simulink model "singlcontact_control_smc_lqr_mydimes_reaction"  (R2024a)
settings: Solver=VariableStepAuto  StartTime=0.0  StopTime=10  FixedStep=0.001  RelTol=1e-3
values from neighbouring files (symbols this model uses):
  ankle_servo_kd = 8    [robotParametersCtrl_mydiem_block_zmp.m]    (also in robotParametersCtrl_quad_modify_mydiem.m; robotParametersCtrl_quad_modify_mydiem_reaction.m)
  ankle_servo_ki = 4    [robotParametersCtrl_mydiem_block_zmp.m]    (also in robotParametersCtrl_quad_modify_mydiem.m; robotParametersCtrl_quad_modify_mydiem_reaction.m)
  ankle_servo_kp = 20    [robotParametersCtrl_mydiem_block_zmp.m]    (also in robotParametersCtrl_quad_modify_mydiem.m; robotParametersCtrl_quad_modify_mydiem_reaction.m)
  deriv_filter_coeff = 100    [robotParametersCtrl_mydiem_block_zmp.m]    (also in robotParametersCtrl_quad_modify_mydiem.m; robotParametersCtrl_quad_modify_mydiem_reaction.m)
  filter_coefficent_pid = 100    [robotParametersCtrl_mydiem_block_zmp.m]    (also in robotParametersCtrl_quad_modify_mydiem.m; robotParametersCtrl_quad_modify_mydiem_reaction.m)
  filter_coefficent_pids = 100    [robotParametersCtrl_quad_modify_mydiem_reaction.m]
  foot_z = 1.5    [robotParametersCtrl_mydiem_block_zmp.m]    (also in robotParametersCtrl_quad_modify_mydiem.m; robotParametersCtrl_quad_modify_mydiem_reaction.m)
  g = 9.81    [ABCDvalues_lqr_quad_mydime_reaction.m]    (also in robotParametersCtrl_mydiem_block_zmp.m = 9.80665; robotParametersCtrl_quad_modify_mydiem.m = 9.80665; robotParametersCtrl_quad_modify_mydiem_reaction.m = 9.80665)
  h = 32    [robotParametersCtrl_mydiem_block_zmp.m]    (also in robotParametersCtrl_quad_modify_mydiem.m; robotParametersCtrl_quad_modify_mydiem_reaction.m)
  height_plane = 0.025    [robotParametersCtrl_mydiem_block_zmp.m]    (also in robotParametersCtrl_quad_modify_mydiem.m; robotParametersCtrl_quad_modify_mydiem_reaction.m)
  hip_pitch_deriv = 20    [robotParametersCtrl_mydiem_block_zmp.m]    (also in robotParametersCtrl_quad_modify_mydiem.m = 200; robotParametersCtrl_quad_modify_mydiem_reaction.m = 200)
  hip_pitch_derivs = 200    [robotParametersCtrl_quad_modify_mydiem_reaction.m]
  hip_pitch_int = 0    [robotParametersCtrl_mydiem_block_zmp.m]    (also in robotParametersCtrl_quad_modify_mydiem.m = 150; robotParametersCtrl_quad_modify_mydiem_reaction.m = 150)
  hip_pitch_ints = 1500    [robotParametersCtrl_quad_modify_mydiem_reaction.m]
  hip_pitch_prop = 10    [robotParametersCtrl_mydiem_block_zmp.m]    (also in robotParametersCtrl_quad_modify_mydiem.m = 500; robotParametersCtrl_quad_modify_mydiem_reaction.m = 500)
  hip_pitch_props = 500    [robotParametersCtrl_quad_modify_mydiem_reaction.m]
  hip_roll_deriv = 28    [robotParametersCtrl_mydiem_block_zmp.m]    (also in robotParametersCtrl_quad_modify_mydiem.m = 280; robotParametersCtrl_quad_modify_mydiem_reaction.m = 280)
  hip_roll_derivs = 280    [robotParametersCtrl_quad_modify_mydiem_reaction.m]
  hip_roll_int = 0    [robotParametersCtrl_mydiem_block_zmp.m]    (also in robotParametersCtrl_quad_modify_mydiem.m = 180; robotParametersCtrl_quad_modify_mydiem_reaction.m = 180)
  hip_roll_ints = 180    [robotParametersCtrl_quad_modify_mydiem_reaction.m]
  hip_roll_prop = 10    [robotParametersCtrl_mydiem_block_zmp.m]    (also in robotParametersCtrl_quad_modify_mydiem.m = 300; robotParametersCtrl_quad_modify_mydiem_reaction.m = 300)
  hip_roll_props = 300    [robotParametersCtrl_quad_modify_mydiem_reaction.m]
  hip_servo_kd = 20    [robotParametersCtrl_mydiem_block_zmp.m]    (also in robotParametersCtrl_quad_modify_mydiem.m; robotParametersCtrl_quad_modify_mydiem_reaction.m)
  hip_servo_ki = 10    [robotParametersCtrl_mydiem_block_zmp.m]    (also in robotParametersCtrl_quad_modify_mydiem.m; robotParametersCtrl_quad_modify_mydiem_reaction.m)
  hip_servo_kp = 60    [robotParametersCtrl_mydiem_block_zmp.m]    (also in robotParametersCtrl_quad_modify_mydiem.m; robotParametersCtrl_quad_modify_mydiem_reaction.m)
  hip_smc_lamda = 85    [robotParametersCtrl_mydiem_block_zmp.m]    (also in robotParametersCtrl_quad_modify_mydiem.m; robotParametersCtrl_quad_modify_mydiem_reaction.m = 95)
  hip_smc_lamdas = 85    [robotParametersCtrl_quad_modify_mydiem_reaction.m]
  hip_smc_new = 25    [robotParametersCtrl_mydiem_block_zmp.m]    (also in robotParametersCtrl_quad_modify_mydiem.m; robotParametersCtrl_quad_modify_mydiem_reaction.m = 45)
  hip_smc_news = 25    [robotParametersCtrl_quad_modify_mydiem_reaction.m]
  init_angs_L = init_angs_R    [robotParametersCtrl_mydiem_block_zmp.m]    (also in robotParametersCtrl_quad_modify_mydiem.m; robotParametersCtrl_quad_modify_mydiem_reaction.m)
  init_angs_R = [0 -sum(init_angs) init_angs(2) 0 init_angs(1)]    [robotParametersCtrl_mydiem_block_zmp.m]    (also in robotParametersCtrl_quad_modify_mydiem.m; robotParametersCtrl_quad_modify_mydiem_reaction.m)
  init_height = h +                torso_z/2 + torso_offset_z + height_plane/2    (= 39.5125)    [robotParametersCtrl_mydiem_block_zmp.m]    (also in robotParametersCtrl_quad_modify_mydiem.m; robotParametersCtrl_quad_modify_mydiem_reaction.m)
  K = lqr(A, B, Q, R)    [ABCDvalues_lqr_quad_mydime_reaction.m]
  knee_pitch_deriv = 10    [robotParametersCtrl_mydiem_block_zmp.m]    (also in robotParametersCtrl_quad_modify_mydiem.m = 100; robotParametersCtrl_quad_modify_mydiem_reaction.m = 100)
  knee_pitch_derivs = 180    [robotParametersCtrl_quad_modify_mydiem_reaction.m]
  knee_pitch_int = 0    [robotParametersCtrl_mydiem_block_zmp.m]    (also in robotParametersCtrl_quad_modify_mydiem.m = 300; robotParametersCtrl_quad_modify_mydiem_reaction.m = 300)
  knee_pitch_ints = 7500    [robotParametersCtrl_quad_modify_mydiem_reaction.m]
  knee_pitch_prop = 10    [robotParametersCtrl_mydiem_block_zmp.m]    (also in robotParametersCtrl_quad_modify_mydiem.m = 400; robotParametersCtrl_quad_modify_mydiem_reaction.m = 400)
  knee_pitch_props = 1200    [robotParametersCtrl_quad_modify_mydiem_reaction.m]
  knee_servo_kd = 10    [robotParametersCtrl_mydiem_block_zmp.m]    (also in robotParametersCtrl_quad_modify_mydiem.m; robotParametersCtrl_quad_modify_mydiem_reaction.m)
  knee_servo_ki = 5    [robotParametersCtrl_mydiem_block_zmp.m]    (also in robotParametersCtrl_quad_modify_mydiem.m; robotParametersCtrl_quad_modify_mydiem_reaction.m)
  knee_servo_kp = 60    [robotParametersCtrl_mydiem_block_zmp.m]    (also in robotParametersCtrl_quad_modify_mydiem.m; robotParametersCtrl_quad_modify_mydiem_reaction.m)
  knee_smc_lamda = 140    [robotParametersCtrl_mydiem_block_zmp.m]    (also in robotParametersCtrl_quad_modify_mydiem.m; robotParametersCtrl_quad_modify_mydiem_reaction.m = 150)
  knee_smc_lamdas = 100    [robotParametersCtrl_quad_modify_mydiem_reaction.m]
  knee_smc_new = 80    [robotParametersCtrl_mydiem_block_zmp.m]    (also in robotParametersCtrl_quad_modify_mydiem.m; robotParametersCtrl_quad_modify_mydiem_reaction.m)
  knee_smc_news = 60    [robotParametersCtrl_quad_modify_mydiem_reaction.m]
  Kwalk = 0.6    [robotParametersCtrl_mydiem_block_zmp.m]    (also in robotParametersCtrl_quad_modify_mydiem.m; robotParametersCtrl_quad_modify_mydiem_reaction.m)
  l1 = 0.20    (= 0.2)    [ABCDvalues_lqr_quad_mydime_reaction.m]
  l2 = 0.20    (= 0.2)    [ABCDvalues_lqr_quad_mydime_reaction.m]
  lower_leg_length = 20    [robotParametersCtrl_mydiem_block_zmp.m]    (also in robotParametersCtrl_quad_modify_mydiem.m; robotParametersCtrl_quad_modify_mydiem_reaction.m)
  m1 = 0.45    [ABCDvalues_lqr_quad_mydime_reaction.m]
  m2 = 0.065    [ABCDvalues_lqr_quad_mydime_reaction.m]
  max_torque = 20    [robotParametersCtrl_mydiem_block_zmp.m]    (also in robotParametersCtrl_quad_modify_mydiem.m; robotParametersCtrl_quad_modify_mydiem_reaction.m)
  motion_time_constant = 0.01    [robotParametersCtrl_mydiem_block_zmp.m]    (also in robotParametersCtrl_quad_modify_mydiem.m; robotParametersCtrl_quad_modify_mydiem_reaction.m)
  plane_x = 25    [robotParametersCtrl_mydiem_block_zmp.m]    (also in robotParametersCtrl_quad_modify_mydiem.m; robotParametersCtrl_quad_modify_mydiem_reaction.m)
  plane_y = 3    [robotParametersCtrl_mydiem_block_zmp.m]    (also in robotParametersCtrl_quad_modify_mydiem.m; robotParametersCtrl_quad_modify_mydiem_reaction.m)
  stepHeight = 0.4    [ABCDvalues_lqr_quad_mydime_reaction.m]
  torso_offset_x = 17    [robotParametersCtrl_mydiem_block_zmp.m]    (also in robotParametersCtrl_quad_modify_mydiem.m; robotParametersCtrl_quad_modify_mydiem_reaction.m)
  torso_offset_x1 = -17    [robotParametersCtrl_mydiem_block_zmp.m]    (also in robotParametersCtrl_quad_modify_mydiem.m; robotParametersCtrl_quad_modify_mydiem_reaction.m)
  torso_offset_z = 0    [robotParametersCtrl_mydiem_block_zmp.m]    (also in robotParametersCtrl_quad_modify_mydiem.m; robotParametersCtrl_quad_modify_mydiem_reaction.m)
  torso_x = 40    [robotParametersCtrl_mydiem_block_zmp.m]    (also in robotParametersCtrl_quad_modify_mydiem.m; robotParametersCtrl_quad_modify_mydiem_reaction.m)
  torso_y = 20    [robotParametersCtrl_mydiem_block_zmp.m]    (also in robotParametersCtrl_quad_modify_mydiem.m; robotParametersCtrl_quad_modify_mydiem_reaction.m)
  torso_z = 15    [robotParametersCtrl_mydiem_block_zmp.m]    (also in robotParametersCtrl_quad_modify_mydiem.m; robotParametersCtrl_quad_modify_mydiem_reaction.m)
  Ts = 0.05    [ABCDvalues_lqr_quad_mydime_reaction.m]
  TsCtrl = 0.05    [robotParametersCtrl_mydiem_block_zmp.m]    (also in robotParametersCtrl_quad_modify_mydiem.m; robotParametersCtrl_quad_modify_mydiem_reaction.m)
  tWalk = 0.3    [robotParametersCtrl_mydiem_block_zmp.m]    (also in robotParametersCtrl_quad_modify_mydiem.m; robotParametersCtrl_quad_modify_mydiem_reaction.m)
  upper_leg_length = 20    [robotParametersCtrl_mydiem_block_zmp.m]    (also in robotParametersCtrl_quad_modify_mydiem.m; robotParametersCtrl_quad_modify_mydiem_reaction.m)
undefined symbols (not defined in the file or in its folder): X, Y, Z
libraries: simulink_extras x256, slpidlib x128, sm_lib x71, simulink x43, nesl_utility x35, walkingRobotUtils x21, dspsrcs4 x18, dspobslib x8
(part 20 of 33)

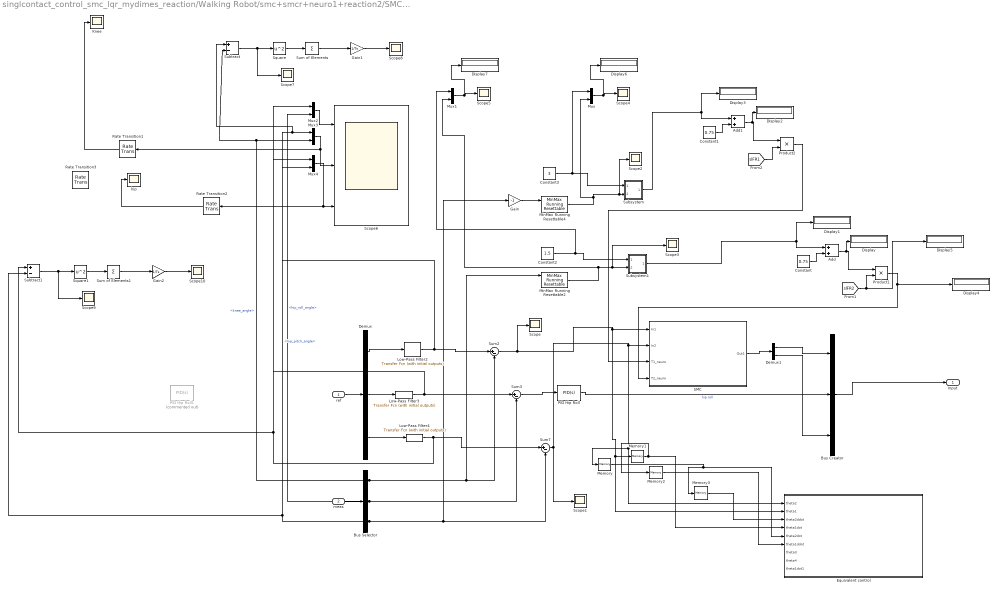
== system singlcontact_control_smc_lqr_mydimes_reaction/Walking Robot/smc+smcr+neuro1+reaction2/SMC Controllers FR4 ==
  ref : Inport
  meas : Inport  Port=2
  Add : Sum
  Add1 : Sum
  Bus Creator : BusCreator  Inputs=3
  Bus Selector : BusSelector  OutputSignals=knee_angle,hip_roll_angle,hip_pitch_angle
  Constant : Constant  Value=0.75
  Constant1 : Constant  Value=0.75
  Constant2 : Constant  Value=1.5
  Constant3 : Constant  Value=3
  Demux : Demux  Outputs=3
  Demux1 : Demux  Outputs=2
  Display{,1..7} (8 alike) : Display
  Equivalent control : Subsystem
  Gain : Gain  Gain=-1
  Gain1 : Gain  Gain=1/Ts
  Gain2 : Gain  Gain=1/Ts
  Knee : Scope
  Low-Pass Filter2 : simulink_extras/Additional Linear/Transfer Fcn (with initial outputs)  N=[(1/motion_time_constant)^2]  D=[1 2/motion_time_constant (1/motion_time_constant)^2]  Y0=init_angs_R(3)  U0=init_angs_R(3)
  Low-Pass Filter3 : simulink_extras/Additional Linear/Transfer Fcn (with initial outputs)  N=[(1/motion_time_constant)^2]  D=[1 2/motion_time_constant (1/motion_time_constant)^2]  Y0=init_angs_R(4)  U0=init_angs_R(4)
  Low-Pass Filter4 : simulink_extras/Additional Linear/Transfer Fcn (with initial outputs)  N=[(1/motion_time_constant)^2]  D=[1 2/motion_time_constant (1/motion_time_constant)^2]  Y0=init_angs_R(5)  U0=init_angs_R(5)
  Memory{,1..3} (4 alike) : Memory
  MinMax Running Resettable2 : simulink/Math Operations/MinMax Running Resettable  Function=max  vinit=0.0
  MinMax Running Resettable4 : simulink/Math Operations/MinMax Running Resettable  Function=max  vinit=0.0
  Mux{,1..4} (5 alike) : Mux  Inputs=2
  PID Hip Roll : slpidlib/PID Controller  Controller=PID  Form=Parallel  TimeDomain=Continuous-time  UseExternalTs=off  SampleTime=-1  IntegratorMethod=Forward Euler  FilterMethod=Forward Euler  ControllerParametersSource=internal  P=hip_roll_prop  I=hip_roll_int  UseKiTs=off  D=hip_roll_deriv  N=filter_coefficent_pid  UseFilter=on  TunerSelectOption=Transfer Function Based (PID Tuner App)  ZeroCross=off  InitialConditionSource=internal  InitialConditionForIntegrator=0  InitialConditionForFilter=0  DifferentiatorICPrevScaledInput=0  ExternalReset=none  TrackingMode=off  Kt=1  LimitOutput=on  SatLimitsSource=internal  UpperSaturationLimit=max_torque  LowerSaturationLimit=-max_torque  LinearizeAsGain=on  AntiWindupMode=clamping  Kb=1  LimitIntegrator=off  UpperIntegratorSaturationLimit=inf  LowerIntegratorSaturationLimit=-inf  POutMin=[]  POutMax=[]  IOutMin=[]  IOutMax=[]  DOutMin=[]  DOutMax=[]  NOutMin=[]  NOutMax=[]  SumOutMin=[]  SumOutMax=[]  SaturationOutMin=[]  SaturationOutMax=[]  PParamMin=[]  PParamMax=[]  IParamMin=[]  IParamMax=[]  DParamMin=[]  DParamMax=[]  NParamMin=[]  NParamMax=[]  KbParamMin=[]  KbParamMax=[]  KtParamMin=[]  KtParamMax=[]  KbOutMin=[]  KbOutMax=[]  KtOutMin=[]  KtOutMax=[]  IntegratorOutMin=[]  IntegratorOutMax=[]  FilterOutMin=[]  FilterOutMax=[]  SumI1OutMin=[]  SumI1OutMax=[]  SumI2OutMin=[]  SumI2OutMax=[]  SumI3OutMin=[]  SumI3OutMax=[]  SumI4OutMin=[]  SumI4OutMax=[]  SumDOutMin=[]  SumDOutMax=[]  DifferentiatorOutMin=[]  DifferentiatorOutMax=[]  FilterDiffOutCoefMin=[]  FilterDiffOutCoefMax=[]  ReciprocalOutMin=[]  ReciprocalOutMax=[]  SumDenOutMin=[]  SumDenOutMax=[]  SumNumOutMin=[]  SumNumOutMax=[]  DivideOutMin=[]  DivideOutMax=[]  UdiffTsProdOutMin=[]  UdiffTsProdOutMax=[]  NTsProdOutMin=[]  NTsProdOutMax=[]  UintegralTsProdOutMin=[]  UintegralTsProdOutMax=[]  UngainTsProdOutMin=[]  UngainTsProdOutMax=[]  ClampingZeroOutDataTypeStr=Inherit: Inherit via back propagation  ClampingZeroOutMin=[]  ClampingZeroOutMax=[]  FilterDenConstantOutDataTypeStr=Inherit: Inherit via back propagation  FilterDenConstantOutMin=[]  FilterDenConstantOutMax=[]  PCopyOutDataTypeStr=Inherit: Inherit via back propagation  PCopyOutMin=[]  PCopyOutMax=[]  NCopyOutDataTypeStr=Inherit: Inherit via back propagation  NCopyOutMin=[]  NCopyOutMax=[]  IntegratorContinuousStateAttributes=''  IntegratorStateMustResolveToSignalObject=off  IntegratorRTWStateStorageClass=Auto  FilterContinuousStateAttributes=''  FilterStateMustResolveToSignalObject=off  FilterRTWStateStorageClass=Auto  ParallelPVariant=InternalParameters  IdealPVariant=Disabled  IVariant=InternalParameters  DVariant=InternalParameters  IntegratorVariant=Continuous  SatVariant=Enabled  AWVariant=ContClampingParallel  PCopyVariant=Disabled  TRVariant=Disabled  FdbkBlocksVariant=Forward  IdealPFdbkVariant=Disabled  SatFdbkVariant=Disabled  DerivativeFilterVariant=ContFilter  NVariant=InternalParameters  NCopyVariant=Disabled  FilterICVariant=InternalICsFilter  IntegratorICVariant=InternalICs  ExternalResetVariant=Disabled  TRSumVariant=Passthrough  SumFdbkVariant=Disabled  SumVariant=Sum_PID  TsampFilterVariant=InternalTs  TsampNgainVariant=Passthrough  TsampIntegralVariant=Disabled_SignalSpec  ExternalSaturationOutDataTypeStr=Inherit: Same as second input
  PID Hip Roll1 : slpidlib/PID Controller  Commented=on  Controller=PID  Form=Parallel  TimeDomain=Continuous-time  UseExternalTs=off  SampleTime=-1  IntegratorMethod=Forward Euler  FilterMethod=Forward Euler  ControllerParametersSource=internal  P=hip_servo_kp  I=hip_servo_ki  UseKiTs=off  D=hip_servo_kd  N=deriv_filter_coeff  UseFilter=on  TunerSelectOption=Transfer Function Based (PID Tuner App)  ZeroCross=off  InitialConditionSource=internal  InitialConditionForIntegrator=0  InitialConditionForFilter=0  DifferentiatorICPrevScaledInput=0  ExternalReset=none  TrackingMode=off  Kt=1  LimitOutput=on  SatLimitsSource=internal  UpperSaturationLimit=max_torque  LowerSaturationLimit=-max_torque  LinearizeAsGain=on  AntiWindupMode=clamping  Kb=1  LimitIntegrator=off  UpperIntegratorSaturationLimit=inf  LowerIntegratorSaturationLimit=-inf  POutMin=[]  POutMax=[]  IOutMin=[]  IOutMax=[]  DOutMin=[]  DOutMax=[]  NOutMin=[]  NOutMax=[]  SumOutMin=[]  SumOutMax=[]  SaturationOutMin=[]  SaturationOutMax=[]  PParamMin=[]  PParamMax=[]  IParamMin=[]  IParamMax=[]  DParamMin=[]  DParamMax=[]  NParamMin=[]  NParamMax=[]  KbParamMin=[]  KbParamMax=[]  KtParamMin=[]  KtParamMax=[]  KbOutMin=[]  KbOutMax=[]  KtOutMin=[]  KtOutMax=[]  IntegratorOutMin=[]  IntegratorOutMax=[]  FilterOutMin=[]  FilterOutMax=[]  SumI1OutMin=[]  SumI1OutMax=[]  SumI2OutMin=[]  SumI2OutMax=[]  SumI3OutMin=[]  SumI3OutMax=[]  SumI4OutMin=[]  SumI4OutMax=[]  SumDOutMin=[]  SumDOutMax=[]  DifferentiatorOutMin=[]  DifferentiatorOutMax=[]  FilterDiffOutCoefMin=[]  FilterDiffOutCoefMax=[]  ReciprocalOutMin=[]  ReciprocalOutMax=[]  SumDenOutMin=[]  SumDenOutMax=[]  SumNumOutMin=[]  SumNumOutMax=[]  DivideOutMin=[]  DivideOutMax=[]  UdiffTsProdOutMin=[]  UdiffTsProdOutMax=[]  NTsProdOutMin=[]  NTsProdOutMax=[]  UintegralTsProdOutMin=[]  UintegralTsProdOutMax=[]  UngainTsProdOutMin=[]  UngainTsProdOutMax=[]  ClampingZeroOutDataTypeStr=Inherit: Inherit via back propagation  ClampingZeroOutMin=[]  ClampingZeroOutMax=[]  FilterDenConstantOutDataTypeStr=Inherit: Inherit via back propagation  FilterDenConstantOutMin=[]  FilterDenConstantOutMax=[]  PCopyOutDataTypeStr=Inherit: Inherit via back propagation  PCopyOutMin=[]  PCopyOutMax=[]  NCopyOutDataTypeStr=Inherit: Inherit via back propagation  NCopyOutMin=[]  NCopyOutMax=[]  IntegratorContinuousStateAttributes=''  IntegratorStateMustResolveToSignalObject=off  IntegratorRTWStateStorageClass=Auto  FilterContinuousStateAttributes=''  FilterStateMustResolveToSignalObject=off  FilterRTWStateStorageClass=Auto  ParallelPVariant=InternalParameters  IdealPVariant=Disabled  IVariant=InternalParameters  DVariant=InternalParameters  IntegratorVariant=Continuous  SatVariant=Enabled  AWVariant=ContClampingParallel  PCopyVariant=Disabled  TRVariant=Disabled  FdbkBlocksVariant=Forward  IdealPFdbkVariant=Disabled  SatFdbkVariant=Disabled  DerivativeFilterVariant=ContFilter  NVariant=InternalParameters  NCopyVariant=Disabled  FilterICVariant=InternalICsFilter  IntegratorICVariant=InternalICs  ExternalResetVariant=Disabled  TRSumVariant=Passthrough  SumFdbkVariant=Disabled  SumVariant=Sum_PID  TsampFilterVariant=InternalTs  TsampNgainVariant=Passthrough  TsampIntegralVariant=Disabled_SignalSpec  ExternalSaturationOutDataTypeStr=Inherit: Same as second input
  Product1 : Product
  Product2 : Product
  Rate Transition1 : RateTransition  OutPortSampleTime=0.005
  Rate Transition2 : RateTransition  OutPortSampleTime=0.005
  Rate Transition3 : RateTransition  OutPortSampleTime=0.005
  SMC : Subsystem
  Scope{,1..5,7..10} (10 alike) : Scope
  Scope6 : Scope  NumInputPorts=3
  Square : Math  Operator=square
  Square1 : Math  Operator=square
  Subsystem : Subsystem
  Subsystem1 : Subsystem
  Subtract : Sum  Inputs=+-
  Subtract1 : Sum  Inputs=+-
  Sum of Elements : Sum  Inputs=+
  Sum of Elements1 : Sum  Inputs=+
  Sum2 : Sum  Inputs=|+-
  Sum3 : Sum  Inputs=|+-
  Sum7 : Sum  Inputs=|+-
  hip : Scope
  Input : Outport  VectorParamsAs1DForOutWhenUnconnected=off
  wires:
  Demux/3 -> Low-Pass Filter4/1
  Demux/1 -> Low-Pass Filter2/1
  Bus Selector/1 -> Mux3/2, Subtract/2, MinMax Running Resettable2/1, Sum2/2  "<knee_angle>"
  Sum7/1 -> Memory/1, Equivalent control/1(theta2), SMC/2(In2), Scope1/1
  Sum3/1 -> PID Hip Roll/1
  ref/1 -> Demux/1
  Sum2/1 -> Scope/1, Memory1/1, Equivalent control/2(theta1), SMC/1(In1)
  Demux/2 -> Low-Pass Filter3/1
  PID Hip Roll/1 -> Bus Creator/2  "hip roll"
  Bus Creator/1 -> Input/1
  Low-Pass Filter2/1 -> Subtract/1, Mux3/1, Sum2/1
  Bus Selector/2 -> Mux2/2, Sum3/2  "<hip_roll_angle>"
  meas/1 -> Bus Selector/1
  Memory/1 -> Equivalent control/5(theta2dot), Memory3/1
  Memory1/1 -> Memory2/1, Equivalent control/4(theta1dot)
  Memory2/1 -> Equivalent control/6(theta1ddot)
  Memory3/1 -> Equivalent control/3(theta2ddot)
  SMC/1(Out1) -> Demux1/1
  Demux1/1 -> Bus Creator/1
  Demux1/2 -> Bus Creator/3
  Constant3/1 -> Mux/1, Subsystem/1(In1)
  MinMax Running Resettable4/1 -> Mux/2, Scope2/1, Subsystem/2(In2)
  Product1/1 -> SMC/4(T2_neuro), Display4/1
  Constant/1 -> Add/2
  Add/1 -> Display/1, Product1/1
  [slFR2] -> Display5/1, Product1/2
  Subsystem1/1(Out1) -> Display1/1, Add/1
  Product2/1 -> SMC/3(T1_neuro)
  Constant1/1 -> Add1/2
  [slFR1] -> Product2/2
  Add1/1 -> Display2/1, Product2/1
  Subsystem/1(Out1) -> Display3/1, Add1/1
  Gain/1 -> MinMax Running Resettable4/1
  Mux/1 -> Display6/1, Scope4/1
  Mux1/1 -> Scope5/1, Display7/1
  MinMax Running Resettable2/1 -> Mux1/2, Scope3/1, Subsystem1/2(In2)
  Constant2/1 -> Mux1/1, Subsystem1/1(In1)
  Low-Pass Filter3/1 -> Mux2/1, Sum3/1
  Mux2/1 -> Scope6/1
  Mux3/1 -> Rate Transition1/1, Scope6/2
  Mux4/1 -> Rate Transition2/1, Scope6/3
  Rate Transition1/1 -> Knee/1
  Rate Transition2/1 -> hip/1
  Subtract/1 -> Scope7/1, Square/1
  Square/1 -> Sum of Elements/1
  Gain1/1 -> Scope8/1
  Sum of Elements/1 -> Gain1/1
  Square1/1 -> Sum of Elements1/1
  Sum of Elements1/1 -> Gain2/1
  Gain2/1 -> Scope10/1
  Bus Selector/3 -> Sum7/2, Gain/1, Subtract1/2, Mux4/2  "<hip_pitch_angle>"
  Low-Pass Filter4/1 -> Subtract1/1, Mux4/1, Sum7/1
  Subtract1/1 -> Scope9/1, Square1/1

== system singlcontact_control_smc_lqr_mydimes_reaction/Walking Robot/smc+smcr+neuro1+reaction2/smc ==
  In1 : Inport
  Enable : EnablePort  StatesWhenEnabling=reset  PropagateVarSize=During execution
  Out1 : Outport
  wires:
  In1/1 -> Out1/1

== system singlcontact_control_smc_lqr_mydimes_reaction/Walking Robot/Lqr+Lqr+reaction/LQR2 Controllers BL/Subsystem2 ==
  <knee_angle> : Inport
  <hip_pitch_angle> : Inport  Port=2
  Gain3 : Gain  Gain=0.5
  Product : Product
  Product3 : Product
  length from ground : Subsystem
  Input : Outport
  Input1 : Outport  Port=2
  wires:
  length from ground/1(Output) -> Product/1
  <knee_angle>/1 -> length from ground/1(In1)
  <hip_pitch_angle>/1 -> length from ground/2(In2)
  [Rbl] -> Gain3/1
  Gain3/1 -> Product3/2, Product/2
  length from ground/2(Outport) -> Product3/1
  Product/1 -> Input/1
  Product3/1 -> Input1/1

== system singlcontact_control_smc_lqr_mydimes_reaction/Walking Robot/Lqr+Lqr+reaction/LQR2 Controllers BR/Subsystem2 ==
  <knee_angle> : Inport
  <hip_pitch_angle> : Inport  Port=2
  Gain3 : Gain  Gain=0.5
  Product : Product
  Product3 : Product
  length from ground : Subsystem
  Input : Outport
  Input1 : Outport  Port=2
  wires:
  Product/1 -> Input/1
  length from ground/2(Outport) -> Product3/1
  Gain3/1 -> Product/2, Product3/2
  Product3/1 -> Input1/1
  [Rbr] -> Gain3/1
  <hip_pitch_angle>/1 -> length from ground/2(In2)
  <knee_angle>/1 -> length from ground/1(In1)
  length from ground/1(Output) -> Product/1

== system singlcontact_control_smc_lqr_mydimes_reaction/Walking Robot/Lqr+Lqr+reaction/LQR2 Controllers FL/Subsystem2 ==
  <knee_angle> : Inport
  <hip_pitch_angle> : Inport  Port=2
  Gain3 : Gain  Gain=0.5
  Product : Product
  Product3 : Product
  length from ground : Subsystem
  Input : Outport
  Input1 : Outport  Port=2
  wires:
  length from ground/1(Output) -> Product/1
  <knee_angle>/1 -> length from ground/1(In1)
  <hip_pitch_angle>/1 -> length from ground/2(In2)
  [Rfl] -> Gain3/1
  Product3/1 -> Input1/1
  Gain3/1 -> Product3/2, Product/2
  length from ground/2(Outport) -> Product3/1
  Product/1 -> Input/1

== system singlcontact_control_smc_lqr_mydimes_reaction/Walking Robot/Lqr+Lqr+reaction/LQR2 Controllers FR/Subsystem2 ==
  <knee_angle> : Inport
  <hip_pitch_angle> : Inport  Port=2
  Gain3 : Gain  Gain=0.5
  Product : Product
  Product3 : Product
  length from ground : Subsystem
  Input : Outport
  Input1 : Outport  Port=2
  wires:
  Product/1 -> Input/1
  length from ground/2(Outport) -> Product3/1
  Gain3/1 -> Product/2, Product3/2
  Product3/1 -> Input1/1
  [Rfr] -> Gain3/1
  <hip_pitch_angle>/1 -> length from ground/2(In2)
  <knee_angle>/1 -> length from ground/1(In1)
  length from ground/1(Output) -> Product/1

== system singlcontact_control_smc_lqr_mydimes_reaction/Walking Robot/Lqr+Lqr+reaction/SMC Controllers FR1/Equivalent control ==
  theta2 : Inport
  theta1 : Inport  Port=2
  theta2ddot : Inport  Port=3
  theta1dot : Inport  Port=4
  theta2dot : Inport  Port=5
  theta1ddot : Inport  Port=6
  theta3 : Inport  Port=7
  theta4 : Inport  Port=8
  theta1dot1 : Inport  Port=9
  Constant : Constant  Value=0
  Constant1 : Constant  Value=0
  SMC equivalent T1 : Subsystem
  SMC equivalent T2 : Subsystem
  Scope : Scope  NumInputPorts=2
  tag scope: TT1FL=global, TT2FL=global
  wires:
  theta1dot1/1 -> SMC equivalent T2/5(theta1dot)
  theta2dot/1 -> SMC equivalent T1/5(theta2dot)
  theta1ddot/1 -> SMC equivalent T2/1(theta1ddot)
  theta4/1 -> SMC equivalent T2/3(theta1)
  theta1/1 -> SMC equivalent T1/2(theta1)
  theta3/1 -> SMC equivalent T2/2(theta2)
  Constant/1 -> SMC equivalent T1/6(theta1ddot)
  theta1dot/1 -> SMC equivalent T1/4(theta1dot)
  theta2ddot/1 -> SMC equivalent T1/3(theta2ddot)
  Constant1/1 -> SMC equivalent T2/4(theta2ddot)
  SMC equivalent T1/1(T1) -> [TT1FL], Scope/2
  theta2/1 -> SMC equivalent T1/1(theta2)
  SMC equivalent T2/1(T2) -> [TT2FL], Scope/1

== system singlcontact_control_smc_lqr_mydimes_reaction/Walking Robot/Lqr+Lqr+reaction/SMC Controllers FR1/SMC ==
  In1 : Inport
  In2 : Inport  Port=2
  T1_neuro : Inport  Port=3
  T2_neuro : Inport  Port=4
  Add : Sum
  Add1 : Sum
  Edot : Derivative
  Edot1 : Derivative
  Gain : Gain  Gain=-0.9
  Gain1 : Gain  Gain=-0.9
  Mux : Mux  Inputs=2
  New : Gain  Gain=25
  New1 : Gain  Gain=25
  Product : Product
  Product2 : Product
  S : Sum
  S1 : Sum
  Scope : Scope  NumInputPorts=2
  Scope{2..5} (4 alike) : Scope
  Sum : Sum  Inputs=++++
  Sum1 : Sum  Inputs=++++
  Tanh : Trigonometry  Operator=tanh
  Tanh1 : Trigonometry  Operator=tanh
  lamda : Constant  Value=50
  lamda1 : Constant  Value=50
  Out1 : Outport
  tag scope: edotFL1=global, edotFL2=global, lamdaFL1=global, lamdaFL2=global
  wires:
  Add1/1 -> Gain1/1
  Gain1/1 -> ?
  Gain/1 -> ?
  Add/1 -> Gain/1
  S/1 -> Tanh1/1
  T2_neuro/1 -> ?
  T1_neuro/1 -> ?
  Sum1/1 -> Scope2/1, Mux/2, Scope4/1
  Sum/1 -> Mux/1, Scope5/1, Scope3/1
  Mux/1 -> Out1/1
  [TT2FL] -> Sum1/2, Add1/2
  [TT1FL] -> Sum/2, Add/2, Scope/2
  New/1 -> Scope/1, Add/1, Sum/1
  Tanh/1 -> New1/1
  lamda/1 -> Product/1, [lamdaFL1]
  Tanh1/1 -> New/1
  Edot1/1 -> [edotFL2], S1/1
  In1/1 -> Product/2, Edot/1
  Product2/1 -> S1/2
  New1/1 -> Sum1/1, Add1/1
  In2/1 -> Edot1/1, Product2/2
  lamda1/1 -> Product2/1, [lamdaFL2]
  Product/1 -> S/2
  Edot/1 -> S/1, [edotFL1]
  S1/1 -> Tanh/1

== system singlcontact_control_smc_lqr_mydimes_reaction/Walking Robot/Lqr+Lqr+reaction/SMC Controllers FR2/Equivalent control ==
  theta2 : Inport
  theta1 : Inport  Port=2
  theta2ddot : Inport  Port=3
  theta1dot : Inport  Port=4
  theta2dot : Inport  Port=5
  theta1ddot : Inport  Port=6
  theta3 : Inport  Port=7
  theta4 : Inport  Port=8
  theta1dot1 : Inport  Port=9
  Constant : Constant  Value=0
  Constant1 : Constant  Value=0
  SMC equivalent T1 : Subsystem
  SMC equivalent T2 : Subsystem
  Scope : Scope  NumInputPorts=2
  tag scope: TT1BR=global, TT2BR=global
  wires:
  SMC equivalent T2/1(T2) -> Scope/1, [TT2BR]
  theta2/1 -> SMC equivalent T1/1(theta2)
  SMC equivalent T1/1(T1) -> Scope/2, [TT1BR]
  Constant1/1 -> SMC equivalent T2/4(theta2ddot)
  theta2ddot/1 -> SMC equivalent T1/3(theta2ddot)
  theta1dot/1 -> SMC equivalent T1/4(theta1dot)
  Constant/1 -> SMC equivalent T1/6(theta1ddot)
  theta3/1 -> SMC equivalent T2/2(theta2)
  theta1/1 -> SMC equivalent T1/2(theta1)
  theta4/1 -> SMC equivalent T2/3(theta1)
  theta1ddot/1 -> SMC equivalent T2/1(theta1ddot)
  theta2dot/1 -> SMC equivalent T1/5(theta2dot)
  theta1dot1/1 -> SMC equivalent T2/5(theta1dot)

== system singlcontact_control_smc_lqr_mydimes_reaction/Walking Robot/Lqr+Lqr+reaction/SMC Controllers FR2/SMC ==
  In1 : Inport
  In2 : Inport  Port=2
  T1_neuro : Inport  Port=3
  T2_neuro : Inport  Port=4
  Add : Sum
  Add1 : Sum
  Edot : Derivative
  Edot1 : Derivative
  Gain : Gain  Gain=-0.9
  Gain1 : Gain  Gain=-0.9
  Mux : Mux  Inputs=2
  New : Gain  Gain=25
  New1 : Gain  Gain=25
  Product : Product
  Product2 : Product
  S : Sum
  S1 : Sum
  Scope : Scope  NumInputPorts=2
  Scope{2..5} (4 alike) : Scope
  Sum : Sum  Inputs=++++
  Sum1 : Sum  Inputs=++++
  Tanh : Trigonometry  Operator=tanh
  Tanh1 : Trigonometry  Operator=tanh
  lamda : Constant  Value=50
  lamda1 : Constant  Value=50
  Out1 : Outport
  tag scope: edotBR1=global, edotBR2=global, lamdaBR1=global, lamdaBR2=global
  wires:
  S1/1 -> Tanh/1
  Edot/1 -> [edotBR1], S/1
  Product/1 -> S/2
  lamda1/1 -> [lamdaBR2], Product2/1
  In2/1 -> Product2/2, Edot1/1
  New1/1 -> Add1/1, Sum1/1
  Product2/1 -> S1/2
  In1/1 -> Edot/1, Product/2
  Edot1/1 -> S1/1, [edotBR2]
  Tanh1/1 -> New/1
  lamda/1 -> [lamdaBR1], Product/1
  Tanh/1 -> New1/1
  New/1 -> Sum/1, Add/1, Scope/1
  [TT1BR] -> Scope/2, Add/2, Sum/2
  [TT2BR] -> Add1/2, Sum1/2
  Mux/1 -> Out1/1
  Sum/1 -> Scope3/1, Scope5/1, Mux/1
  Sum1/1 -> Scope4/1, Mux/2, Scope2/1
  T1_neuro/1 -> ?
  T2_neuro/1 -> ?
  S/1 -> Tanh1/1
  Add/1 -> Gain/1
  Gain/1 -> ?
  Gain1/1 -> ?
  Add1/1 -> Gain1/1

== system singlcontact_control_smc_lqr_mydimes_reaction/Walking Robot/Lqr+Lqr+reaction/SMC Controllers FR3/Equivalent control ==
  theta2 : Inport
  theta1 : Inport  Port=2
  theta2ddot : Inport  Port=3
  theta1dot : Inport  Port=4
  theta2dot : Inport  Port=5
  theta1ddot : Inport  Port=6
  theta3 : Inport  Port=7
  theta4 : Inport  Port=8
  theta1dot1 : Inport  Port=9
  Constant : Constant  Value=0
  Constant1 : Constant  Value=0
  SMC equivalent T1 : Subsystem
  SMC equivalent T2 : Subsystem
  Scope : Scope  NumInputPorts=2
  tag scope: TT1BL=global, TT2BL=global
  wires:
  theta1dot1/1 -> SMC equivalent T2/5(theta1dot)
  theta2dot/1 -> SMC equivalent T1/5(theta2dot)
  theta1ddot/1 -> SMC equivalent T2/1(theta1ddot)
  theta4/1 -> SMC equivalent T2/3(theta1)
  theta1/1 -> SMC equivalent T1/2(theta1)
  theta3/1 -> SMC equivalent T2/2(theta2)
  Constant/1 -> SMC equivalent T1/6(theta1ddot)
  theta1dot/1 -> SMC equivalent T1/4(theta1dot)
  theta2ddot/1 -> SMC equivalent T1/3(theta2ddot)
  Constant1/1 -> SMC equivalent T2/4(theta2ddot)
  SMC equivalent T1/1(T1) -> [TT1BL], Scope/2
  theta2/1 -> SMC equivalent T1/1(theta2)
  SMC equivalent T2/1(T2) -> [TT2BL], Scope/1

== system singlcontact_control_smc_lqr_mydimes_reaction/Walking Robot/Lqr+Lqr+reaction/SMC Controllers FR3/SMC ==
  In1 : Inport
  In2 : Inport  Port=2
  T1_neuro : Inport  Port=3
  T2_neuro : Inport  Port=4
  Add : Sum
  Add1 : Sum
  Edot : Derivative
  Edot1 : Derivative
  Gain : Gain  Gain=-0.9
  Gain1 : Gain  Gain=-0.9
  Mux : Mux  Inputs=2
  New : Gain  Gain=25
  New1 : Gain  Gain=25
  Product : Product
  Product2 : Product
  S : Sum
  S1 : Sum
  Scope : Scope  NumInputPorts=2
  Scope{2..5} (4 alike) : Scope
  Sum : Sum  Inputs=++++
  Sum1 : Sum  Inputs=++++
  Tanh : Trigonometry  Operator=tanh
  Tanh1 : Trigonometry  Operator=tanh
  lamda : Constant  Value=50
  lamda1 : Constant  Value=50
  Out1 : Outport
  tag scope: edotBL1=global, edotBL2=global, lamdaBL1=global, lamdaBL2=global
  wires:
  Add1/1 -> Gain1/1
  Gain1/1 -> ?
  Gain/1 -> ?
  Add/1 -> Gain/1
  S/1 -> Tanh1/1
  T2_neuro/1 -> ?
  T1_neuro/1 -> ?
  Sum1/1 -> Scope2/1, Mux/2, Scope4/1
  Sum/1 -> Mux/1, Scope5/1, Scope3/1
  Mux/1 -> Out1/1
  [TT2BL] -> Sum1/2, Add1/2
  [TT1BL] -> Sum/2, Add/2, Scope/2
  New/1 -> Scope/1, Add/1, Sum/1
  Tanh/1 -> New1/1
  lamda/1 -> Product/1, [lamdaBL1]
  Tanh1/1 -> New/1
  Edot1/1 -> [edotBL2], S1/1
  In1/1 -> Product/2, Edot/1
  Product2/1 -> S1/2
  New1/1 -> Sum1/1, Add1/1
  In2/1 -> Edot1/1, Product2/2
  lamda1/1 -> Product2/1, [lamdaBL2]
  Product/1 -> S/2
  Edot/1 -> S/1, [edotBL1]
  S1/1 -> Tanh/1

== system singlcontact_control_smc_lqr_mydimes_reaction/Walking Robot/Pid+Pid+reaction1/PID Controllers FR4/Subsystem2 ==
  <knee_angle> : Inport
  <hip_pitch_angle> : Inport  Port=2
  Gain3 : Gain  Gain=0.5
  Product : Product
  Product3 : Product
  length from ground : Subsystem
  Input : Outport
  Input1 : Outport  Port=2
  wires:
  Product/1 -> Input/1
  length from ground/2(Outport) -> Product3/1
  Gain3/1 -> Product/2, Product3/2
  Product3/1 -> Input1/1
  [Rfr] -> Gain3/1
  <hip_pitch_angle>/1 -> length from ground/2(In2)
  <knee_angle>/1 -> length from ground/1(In1)
  length from ground/1(Output) -> Product/1

== system singlcontact_control_smc_lqr_mydimes_reaction/Walking Robot/Pid+Pid+reaction1/PID Controllers FR5/Subsystem2 ==
  <knee_angle> : Inport
  <hip_pitch_angle> : Inport  Port=2
  Gain3 : Gain  Gain=0.5
  Product : Product
  Product3 : Product
  length from ground : Subsystem
  Input : Outport
  Input1 : Outport  Port=2
  wires:
  Product/1 -> Input/1
  length from ground/2(Outport) -> Product3/1
  Gain3/1 -> Product/2, Product3/2
  Product3/1 -> Input1/1
  [Rfr] -> Gain3/1
  <hip_pitch_angle>/1 -> length from ground/2(In2)
  <knee_angle>/1 -> length from ground/1(In1)
  length from ground/1(Output) -> Product/1

== system singlcontact_control_smc_lqr_mydimes_reaction/Walking Robot/Pid+Pid+reaction1/PID Controllers FR6/Subsystem2 ==
  <knee_angle> : Inport
  <hip_pitch_angle> : Inport  Port=2
  Gain3 : Gain  Gain=0.5
  Product : Product
  Product3 : Product
  length from ground : Subsystem
  Input : Outport
  Input1 : Outport  Port=2
  wires:
  Product/1 -> Input/1
  length from ground/2(Outport) -> Product3/1
  Gain3/1 -> Product/2, Product3/2
  Product3/1 -> Input1/1
  [Rfr] -> Gain3/1
  <hip_pitch_angle>/1 -> length from ground/2(In2)
  <knee_angle>/1 -> length from ground/1(In1)
  length from ground/1(Output) -> Product/1

== system singlcontact_control_smc_lqr_mydimes_reaction/Walking Robot/Pid+Pid+reaction1/PID Controllers FR7/Subsystem2 ==
  <knee_angle> : Inport
  <hip_pitch_angle> : Inport  Port=2
  Gain3 : Gain  Gain=0.5
  Product : Product
  Product3 : Product
  length from ground : Subsystem
  Input : Outport
  Input1 : Outport  Port=2
  wires:
  Product/1 -> Input/1
  length from ground/2(Outport) -> Product3/1
  Gain3/1 -> Product/2, Product3/2
  Product3/1 -> Input1/1
  [Rfr] -> Gain3/1
  <hip_pitch_angle>/1 -> length from ground/2(In2)
  <knee_angle>/1 -> length from ground/1(In1)
  length from ground/1(Output) -> Product/1

== system singlcontact_control_smc_lqr_mydimes_reaction/Walking Robot/Pid+Pid+reaction1/SMC Controllers FR1/Equivalent control ==
  theta2 : Inport
  theta1 : Inport  Port=2
  theta2ddot : Inport  Port=3
  theta1dot : Inport  Port=4
  theta2dot : Inport  Port=5
  theta1ddot : Inport  Port=6
  theta3 : Inport  Port=7
  theta4 : Inport  Port=8
  theta1dot1 : Inport  Port=9
  Constant : Constant  Value=0
  Constant1 : Constant  Value=0
  SMC equivalent T1 : Subsystem
  SMC equivalent T2 : Subsystem
  Scope : Scope  NumInputPorts=2
  tag scope: TT1FL=global, TT2FL=global
  wires:
  theta1dot1/1 -> SMC equivalent T2/5(theta1dot)
  theta2dot/1 -> SMC equivalent T1/5(theta2dot)
  theta1ddot/1 -> SMC equivalent T2/1(theta1ddot)
  theta4/1 -> SMC equivalent T2/3(theta1)
  theta1/1 -> SMC equivalent T1/2(theta1)
  theta3/1 -> SMC equivalent T2/2(theta2)
  Constant/1 -> SMC equivalent T1/6(theta1ddot)
  theta1dot/1 -> SMC equivalent T1/4(theta1dot)
  theta2ddot/1 -> SMC equivalent T1/3(theta2ddot)
  Constant1/1 -> SMC equivalent T2/4(theta2ddot)
  SMC equivalent T1/1(T1) -> [TT1FL], Scope/2
  theta2/1 -> SMC equivalent T1/1(theta2)
  SMC equivalent T2/1(T2) -> [TT2FL], Scope/1

== system singlcontact_control_smc_lqr_mydimes_reaction/Walking Robot/Pid+Pid+reaction1/SMC Controllers FR1/SMC ==
  In1 : Inport
  In2 : Inport  Port=2
  T1_neuro : Inport  Port=3
  T2_neuro : Inport  Port=4
  Add : Sum
  Add1 : Sum
  Edot : Derivative
  Edot1 : Derivative
  Gain : Gain  Gain=-0.9
  Gain1 : Gain  Gain=-0.9
  Mux : Mux  Inputs=2
  New : Gain  Gain=25
  New1 : Gain  Gain=25
  Product : Product
  Product2 : Product
  S : Sum
  S1 : Sum
  Scope : Scope  NumInputPorts=2
  Scope{2..5} (4 alike) : Scope
  Sum : Sum  Inputs=++++
  Sum1 : Sum  Inputs=++++
  Tanh : Trigonometry  Operator=tanh
  Tanh1 : Trigonometry  Operator=tanh
  lamda : Constant  Value=50
  lamda1 : Constant  Value=50
  Out1 : Outport
  tag scope: edotFL1=global, edotFL2=global, lamdaFL1=global, lamdaFL2=global
  wires:
  Add1/1 -> Gain1/1
  Gain1/1 -> ?
  Gain/1 -> ?
  Add/1 -> Gain/1
  S/1 -> Tanh1/1
  T2_neuro/1 -> ?
  T1_neuro/1 -> ?
  Sum1/1 -> Scope2/1, Mux/2, Scope4/1
  Sum/1 -> Mux/1, Scope5/1, Scope3/1
  Mux/1 -> Out1/1
  [TT2FL] -> Sum1/2, Add1/2
  [TT1FL] -> Sum/2, Add/2, Scope/2
  New/1 -> Scope/1, Add/1, Sum/1
  Tanh/1 -> New1/1
  lamda/1 -> Product/1, [lamdaFL1]
  Tanh1/1 -> New/1
  Edot1/1 -> [edotFL2], S1/1
  In1/1 -> Product/2, Edot/1
  Product2/1 -> S1/2
  New1/1 -> Sum1/1, Add1/1
  In2/1 -> Edot1/1, Product2/2
  lamda1/1 -> Product2/1, [lamdaFL2]
  Product/1 -> S/2
  Edot/1 -> S/1, [edotFL1]
  S1/1 -> Tanh/1

== system singlcontact_control_smc_lqr_mydimes_reaction/Walking Robot/Pid+Pid+reaction1/SMC Controllers FR2/Equivalent control ==
  theta2 : Inport
  theta1 : Inport  Port=2
  theta2ddot : Inport  Port=3
  theta1dot : Inport  Port=4
  theta2dot : Inport  Port=5
  theta1ddot : Inport  Port=6
  theta3 : Inport  Port=7
  theta4 : Inport  Port=8
  theta1dot1 : Inport  Port=9
  Constant : Constant  Value=0
  Constant1 : Constant  Value=0
  SMC equivalent T1 : Subsystem
  SMC equivalent T2 : Subsystem
  Scope : Scope  NumInputPorts=2
  tag scope: TT1BR=global, TT2BR=global
  wires:
  SMC equivalent T2/1(T2) -> Scope/1, [TT2BR]
  theta2/1 -> SMC equivalent T1/1(theta2)
  SMC equivalent T1/1(T1) -> Scope/2, [TT1BR]
  Constant1/1 -> SMC equivalent T2/4(theta2ddot)
  theta2ddot/1 -> SMC equivalent T1/3(theta2ddot)
  theta1dot/1 -> SMC equivalent T1/4(theta1dot)
  Constant/1 -> SMC equivalent T1/6(theta1ddot)
  theta3/1 -> SMC equivalent T2/2(theta2)
  theta1/1 -> SMC equivalent T1/2(theta1)
  theta4/1 -> SMC equivalent T2/3(theta1)
  theta1ddot/1 -> SMC equivalent T2/1(theta1ddot)
  theta2dot/1 -> SMC equivalent T1/5(theta2dot)
  theta1dot1/1 -> SMC equivalent T2/5(theta1dot)

== system singlcontact_control_smc_lqr_mydimes_reaction/Walking Robot/Pid+Pid+reaction1/SMC Controllers FR2/SMC ==
  In1 : Inport
  In2 : Inport  Port=2
  T1_neuro : Inport  Port=3
  T2_neuro : Inport  Port=4
  Add : Sum
  Add1 : Sum
  Edot : Derivative
  Edot1 : Derivative
  Gain : Gain  Gain=-0.9
  Gain1 : Gain  Gain=-0.9
  Mux : Mux  Inputs=2
  New : Gain  Gain=25
  New1 : Gain  Gain=25
  Product : Product
  Product2 : Product
  S : Sum
  S1 : Sum
  Scope : Scope  NumInputPorts=2
  Scope{2..5} (4 alike) : Scope
  Sum : Sum  Inputs=++++
  Sum1 : Sum  Inputs=++++
  Tanh : Trigonometry  Operator=tanh
  Tanh1 : Trigonometry  Operator=tanh
  lamda : Constant  Value=50
  lamda1 : Constant  Value=50
  Out1 : Outport
  tag scope: edotBR1=global, edotBR2=global, lamdaBR1=global, lamdaBR2=global
  wires:
  S1/1 -> Tanh/1
  Edot/1 -> [edotBR1], S/1
  Product/1 -> S/2
  lamda1/1 -> [lamdaBR2], Product2/1
  In2/1 -> Product2/2, Edot1/1
  New1/1 -> Add1/1, Sum1/1
  Product2/1 -> S1/2
  In1/1 -> Edot/1, Product/2
  Edot1/1 -> S1/1, [edotBR2]
  Tanh1/1 -> New/1
  lamda/1 -> [lamdaBR1], Product/1
  Tanh/1 -> New1/1
  New/1 -> Sum/1, Add/1, Scope/1
  [TT1BR] -> Scope/2, Add/2, Sum/2
  [TT2BR] -> Add1/2, Sum1/2
  Mux/1 -> Out1/1
  Sum/1 -> Scope3/1, Scope5/1, Mux/1
  Sum1/1 -> Scope4/1, Mux/2, Scope2/1
  T1_neuro/1 -> ?
  T2_neuro/1 -> ?
  S/1 -> Tanh1/1
  Add/1 -> Gain/1
  Gain/1 -> ?
  Gain1/1 -> ?
  Add1/1 -> Gain1/1

== system singlcontact_control_smc_lqr_mydimes_reaction/Walking Robot/Pid+Pid+reaction1/SMC Controllers FR3/Equivalent control ==
  theta2 : Inport
  theta1 : Inport  Port=2
  theta2ddot : Inport  Port=3
  theta1dot : Inport  Port=4
  theta2dot : Inport  Port=5
  theta1ddot : Inport  Port=6
  theta3 : Inport  Port=7
  theta4 : Inport  Port=8
  theta1dot1 : Inport  Port=9
  Constant : Constant  Value=0
  Constant1 : Constant  Value=0
  SMC equivalent T1 : Subsystem
  SMC equivalent T2 : Subsystem
  Scope : Scope  NumInputPorts=2
  tag scope: TT1BL=global, TT2BL=global
  wires:
  theta1dot1/1 -> SMC equivalent T2/5(theta1dot)
  theta2dot/1 -> SMC equivalent T1/5(theta2dot)
  theta1ddot/1 -> SMC equivalent T2/1(theta1ddot)
  theta4/1 -> SMC equivalent T2/3(theta1)
  theta1/1 -> SMC equivalent T1/2(theta1)
  theta3/1 -> SMC equivalent T2/2(theta2)
  Constant/1 -> SMC equivalent T1/6(theta1ddot)
  theta1dot/1 -> SMC equivalent T1/4(theta1dot)
  theta2ddot/1 -> SMC equivalent T1/3(theta2ddot)
  Constant1/1 -> SMC equivalent T2/4(theta2ddot)
  SMC equivalent T1/1(T1) -> [TT1BL], Scope/2
  theta2/1 -> SMC equivalent T1/1(theta2)
  SMC equivalent T2/1(T2) -> [TT2BL], Scope/1

== system singlcontact_control_smc_lqr_mydimes_reaction/Walking Robot/Pid+Pid+reaction1/SMC Controllers FR3/SMC ==
  In1 : Inport
  In2 : Inport  Port=2
  T1_neuro : Inport  Port=3
  T2_neuro : Inport  Port=4
  Add : Sum
  Add1 : Sum
  Edot : Derivative
  Edot1 : Derivative
  Gain : Gain  Gain=-0.9
  Gain1 : Gain  Gain=-0.9
  Mux : Mux  Inputs=2
  New : Gain  Gain=25
  New1 : Gain  Gain=25
  Product : Product
  Product2 : Product
  S : Sum
  S1 : Sum
  Scope : Scope  NumInputPorts=2
  Scope{2..5} (4 alike) : Scope
  Sum : Sum  Inputs=++++
  Sum1 : Sum  Inputs=++++
  Tanh : Trigonometry  Operator=tanh
  Tanh1 : Trigonometry  Operator=tanh
  lamda : Constant  Value=50
  lamda1 : Constant  Value=50
  Out1 : Outport
  tag scope: edotBL1=global, edotBL2=global, lamdaBL1=global, lamdaBL2=global
  wires:
  Add1/1 -> Gain1/1
  Gain1/1 -> ?
  Gain/1 -> ?
  Add/1 -> Gain/1
  S/1 -> Tanh1/1
  T2_neuro/1 -> ?
  T1_neuro/1 -> ?
  Sum1/1 -> Scope2/1, Mux/2, Scope4/1
  Sum/1 -> Mux/1, Scope5/1, Scope3/1
  Mux/1 -> Out1/1
  [TT2BL] -> Sum1/2, Add1/2
  [TT1BL] -> Sum/2, Add/2, Scope/2
  New/1 -> Scope/1, Add/1, Sum/1
  Tanh/1 -> New1/1
  lamda/1 -> Product/1, [lamdaBL1]
  Tanh1/1 -> New/1
  Edot1/1 -> [edotBL2], S1/1
  In1/1 -> Product/2, Edot/1
  Product2/1 -> S1/2
  New1/1 -> Sum1/1, Add1/1
  In2/1 -> Edot1/1, Product2/2
  lamda1/1 -> Product2/1, [lamdaBL2]
  Product/1 -> S/2
  Edot/1 -> S/1, [edotBL1]
  S1/1 -> Tanh/1
